simulink model "NonAtomicSubsystem"  (R2022b)
settings: Solver=VariableStepAuto  StartTime=0.0  StopTime=10.0  RelTol=1e-3
settings Model: Creator=Brigosha_Guest  LastModifiedBy=Brigosha_Guest

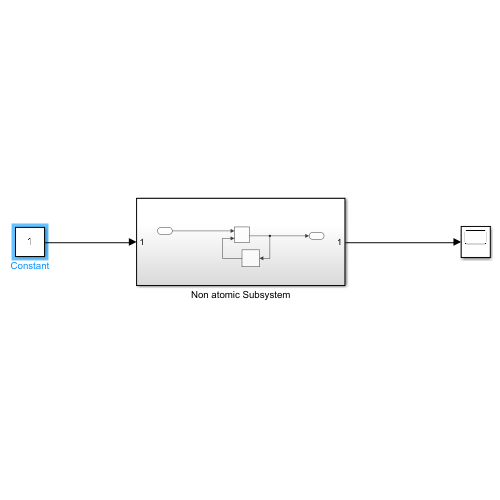
[thumbnail: Simulink's stored preview of the top-level diagram]
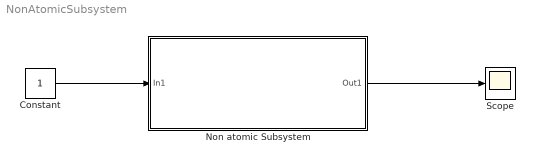
== system NonAtomicSubsystem ==
  Constant : Constant
  Non atomic Subsystem : Subsystem
  Scope : Scope
  wires:
  Constant/1 -> Non atomic Subsystem/1(In1)
  Non atomic Subsystem/1(Out1) -> Scope/1

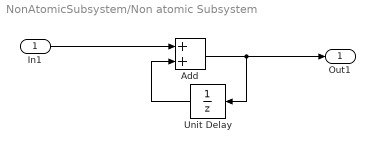
== system NonAtomicSubsystem/Non atomic Subsystem ==
  In1 : Inport
  Add : Sum
  Unit Delay : UnitDelay  SampleTime=-1  HasFrameUpgradeWarning=on
  Out1 : Outport
  wires:
  Unit Delay/1 -> Add/2
  In1/1 -> Add/1
  Add/1 -> Out1/1, Unit Delay/1
